simulink model "gm_soc_dvbs2_fpga"  (R2025b)
settings: Solver=VariableStepAuto  StartTime=0.0  StopTime=10.0  RelTol=1e-3
InitFcn:
  | soc_dvbs2_init;
undefined symbols (not defined in the file or in its folder): Add, coefficientsLog, coefficientsSqrt1, coefficientsSqrt2, dataBits, Deinterleaver, designMultirateFIR, noisePow, Shift, Short, soc_dvbs2_designFIRFilter, soc_dvbs2_txPacketBits, syncWord, txDataOut, txFiltCoeff, XData
libraries: simulink x304, hdlsllib x265, dspsigops x15, dsphdlfiltering2 x8, hdlmdlgenlib x6, dsphdlsigops2 x5, commseqgen3 x5, dsphdlmathfun2 x3, hwlogicconnlib x2, whdledac x2, commhdlcrc x2, whdlutilities x1
(part 8 of 36)

== system gm_soc_dvbs2_fpga/DVBS2/DVBS2 TxRx/Channel/AWGN Generator/Unit Variance Gaussian Noise/SinCos ==
  u1 : Inport  OutDataTypeStr=fixdt(0, 16, 16)  PortDimensions=1  SampleTime=6.25e-08
  Delay : Delay  DelayLength=double(1)  InitialCondition=0  SampleTime=6.25e-08
  Delay1 : Delay  DelayLength=double(1)  InitialCondition=0  SampleTime=6.25e-08
  Delay3 : Delay  DelayLength=double(1)  InitialCondition=0  SampleTime=6.25e-08
  Sine HDL Optimized1 : Subsystem  mask(Sine and Cosine HDL optimized block){OutputFormula=cos(2*pi*u), NumDataPoints=double(1024), TableDataTypeStr=fixdt(0,15,15), SimulateLUTROMDelay=off}
      mask prompts: OutputFormula "Simulink:masks:OutputFormula_MP"; NumDataPoints "HDLShared:hdlshared:CosineHDL_Npts"; TableDataTypeStr "Simulink:blkprm_prompts:TABLE_UNIFIEDDATATYPE"; SimulateLUTROMDelay "HDLShared:hdlshared:CosineHDL_SimulateLUTDelay"
      mask help: Sine and Cosine HDL optimized block using quarter wave symmetry, and HDL friendly settings.
      mask init:
      | NumDataPoints = double(1024);
      | OutputFormula = double(2);
      | SampleTime = double(-1);
      | SimulateLUTROMDelay = double(0);
      | TableDataTypeStr = fixdt(0,15,15);
      | curr_blk_name = 'soc_dvbs2_fpga/DVBS2/DVBS2 TxRx/Channel/AWGN Generator/Unit Variance Gaussian Noise/SinCos/Sine\nHDL Optimized1';
      | sys_name = 'soc_dvbs2_fpga/DVBS2/DVBS2 TxRx/Channel/AWGN Generator/Unit Variance Gaussian Noise/SinCos';
      mask Help: helpview([docroot '/hdlcoder/helptargets.map'],'SineAndCosineHDL_Optimized');
      mask TypeOptions OutputFormula: sin(2*pi*u) | cos(2*pi*u) | exp(j*2*pi*u) | sin(2*pi*u) and cos(2*pi*u)
      mask Display:
      | port_label('input',1,'u')
      | port_label('output',1,'cos(2*pi*u)')
      | xpos = 0.35;
      | yoffset = 0.5;
      | if ( SimulateLUTROMDelay )
      |   text(xpos,yoffset,'HDL (Z^{-1})','texmode','on')
      | else
      |    text(xpos,yoffset,'HDL')
      | end
  Sine HDL Optimized2 : Subsystem  mask(Sine and Cosine HDL optimized block){OutputFormula=sin(2*pi*u), NumDataPoints=double(1024), TableDataTypeStr=fixdt(0,15,15), SimulateLUTROMDelay=off}
      mask prompts: OutputFormula "Simulink:masks:OutputFormula_MP"; NumDataPoints "HDLShared:hdlshared:CosineHDL_Npts"; TableDataTypeStr "Simulink:blkprm_prompts:TABLE_UNIFIEDDATATYPE"; SimulateLUTROMDelay "HDLShared:hdlshared:CosineHDL_SimulateLUTDelay"
      mask help: Sine and Cosine HDL optimized block using quarter wave symmetry, and HDL friendly settings.
      mask init:
      | NumDataPoints = double(1024);
      | OutputFormula = double(1);
      | SampleTime = double(-1);
      | SimulateLUTROMDelay = double(0);
      | TableDataTypeStr = fixdt(0,15,15);
      | curr_blk_name = 'soc_dvbs2_fpga/DVBS2/DVBS2 TxRx/Channel/AWGN Generator/Unit Variance Gaussian Noise/SinCos/Sine\nHDL Optimized2';
      | sys_name = 'soc_dvbs2_fpga/DVBS2/DVBS2 TxRx/Channel/AWGN Generator/Unit Variance Gaussian Noise/SinCos';
      mask Help: helpview([docroot '/hdlcoder/helptargets.map'],'SineAndCosineHDL_Optimized');
      mask TypeOptions OutputFormula: sin(2*pi*u) | cos(2*pi*u) | exp(j*2*pi*u) | sin(2*pi*u) and cos(2*pi*u)
      mask Display:
      | port_label('input',1,'u')
      | port_label('output',1,'sin(2*pi*u)')
      | xpos = 0.35;
      | yoffset = 0.5;
      | if ( SimulateLUTROMDelay )
      |   text(xpos,yoffset,'HDL (Z^{-1})','texmode','on')
      | else
      |    text(xpos,yoffset,'HDL')
      | end
  g0 : Outport  SampleTime=6.25e-08
  g1(16,15) : Outport  Port=2  SampleTime=6.25e-08
  wires:
  Sine HDL Optimized1/1(x) -> Delay1/1
  u1/1 -> Delay3/1
  Delay3/1 -> Sine HDL Optimized2/1(u), Sine HDL Optimized1/1(u)
  Sine HDL Optimized2/1(x) -> Delay/1
  Delay1/1 -> g1(16,15)/1
  Delay/1 -> g0/1

== system gm_soc_dvbs2_fpga/DVBS2/DVBS2 TxRx/Channel/AWGN Generator/Unit Variance Gaussian Noise/SqrtImplementation ==
  u : Inport  OutDataTypeStr=fixdt(0, 31, 24)  PortDimensions=1  SampleTime=6.25e-08
  Constant : Constant  Value=0  OutDataTypeStr=fixdt(0,17,13)  SampleTime=-1
  Delay : Delay  DelayLength=19
  Delay1 : Delay  DelayLength=19
  SqrtEval : Subsystem
  Switch : Switch  Criteria=u2 ~= 0  OutDataTypeStr=fixdt(0, 17, 13)  SaturateOnIntegerOverflow=off  InputSameDT=off
  f : Outport  SampleTime=6.25e-08  VectorParamsAs1DForOutWhenUnconnected=off
  wires:
  u/1 -> Delay/1, SqrtEval/1(u)
  Switch/1 -> f/1
  Delay/1 -> Switch/2
  Constant/1 -> Delay1/1
  Delay1/1 -> Switch/3
  SqrtEval/1(f) -> Switch/1

== system gm_soc_dvbs2_fpga/DVBS2/DVBS2 TxRx/Channel/AWGN Generator/Unit Variance Gaussian Noise/TausUniformRandGen ==
  ConcatandExtract : Subsystem
  TausURNG1 : Subsystem
  TausURNG2 : Subsystem
  u0(16,16) : Outport  SampleTime=6.25e-08
  u1(16,16) : Outport  Port=2  SampleTime=6.25e-08
  wires:
  TausURNG1/1(a) -> ConcatandExtract/1(a)
  TausURNG2/1(b) -> ConcatandExtract/2(b)
  ConcatandExtract/2(u1(16,16)) -> u1(16,16)/1
  ConcatandExtract/1(u0(48,48)) -> u0(16,16)/1

== system gm_soc_dvbs2_fpga/DVBS2/DVBS2 TxRx/Channel/AWGN Generator/Unit Variance Gaussian Noise/logImplementation ==
  u0(48,48) : Inport  OutDataTypeStr=fixdt(0, 48, 48)  PortDimensions=1  SampleTime=6.25e-08
  Constant : Constant  Value=0  OutDataTypeStr=fixdt(0,16,9)  SampleTime=-1
  Delay : Delay  DelayLength=24
  Switch : Switch  Criteria=u2 ~= 0  OutDataTypeStr=fixdt(0, 31, 24)  SaturateOnIntegerOverflow=off  InputSameDT=off
  log : Subsystem
  e : Outport  SampleTime=6.25e-08
  wires:
  u0(48,48)/1 -> Delay/1, log/1(u0(48,48))
  log/1(e) -> Switch/1
  Switch/1 -> e/1
  Constant/1 -> Switch/3
  Delay/1 -> Switch/2

== system gm_soc_dvbs2_fpga/DVBS2/DVBS2 TxRx/DVB-S2 HDL Receiver/Demod Deinterleave and FECDecode/DVBS2 HDL Deinterleaver/Discard Out of  Frame samples ==
  dataIn : Inport  OutDataTypeStr=fixdt(1, 8, 4)  PortDimensions=1  SampleTime=7.8125e-09
  valid : Inport  Port=2  OutDataTypeStr=boolean  PortDimensions=1  SampleTime=7.8125e-09
  reset : Inport  Port=3  OutDataTypeStr=boolean  PortDimensions=1  SampleTime=7.8125e-09
  fec : Inport  Port=4  OutDataTypeStr=boolean  PortDimensions=1  SampleTime=7.8125e-09
  Discard Out of  Frame samples : MATLAB Function  TreatAsAtomicUnit=on
  dataOut : Outport  SampleTime=7.8125e-09
  validOut : Outport  Port=2  SampleTime=7.8125e-09
  wires:
  reset/1 -> Discard Out of  Frame samples/3(reset)
  dataIn/1 -> Discard Out of  Frame samples/1(dataIn)
  valid/1 -> Discard Out of  Frame samples/2(valid)
  fec/1 -> Discard Out of  Frame samples/4(fec)
  Discard Out of  Frame samples/2(validOut) -> validOut/1
  Discard Out of  Frame samples/1(dataOut) -> dataOut/1

== system gm_soc_dvbs2_fpga/DVBS2/DVBS2 TxRx/DVB-S2 HDL Receiver/Demod Deinterleave and FECDecode/DVBS2 HDL Deinterleaver/RAM ==
  wr_din : Inport  OutDataTypeStr=fixdt(1, 8, 4)  PortDimensions=1  SampleTime=7.8125e-09
  wr_addr : Inport  Port=2  OutDataTypeStr=fixdt(0, 17, 0)  PortDimensions=1  SampleTime=7.8125e-09
  wr_en : Inport  Port=3  OutDataTypeStr=boolean  PortDimensions=1  SampleTime=7.8125e-09
  rd_addr : Inport  Port=4  OutDataTypeStr=fixdt(0, 18, 0)  PortDimensions=1  SampleTime=7.8125e-09
  rd_valid : Inport  Port=5  OutDataTypeStr=boolean  PortDimensions=1  SampleTime=7.8125e-09
  rd_end : Inport  Port=6  OutDataTypeStr=boolean  PortDimensions=1  SampleTime=7.8125e-09
  rd_start : Inport  Port=7  OutDataTypeStr=boolean  PortDimensions=1  SampleTime=7.8125e-09
  Delay : Delay  DelayLength=1
  Delay1 : Delay  DelayLength=1
  Delay{3..13} (11 alike) : Delay
  Delay2 : Delay  DelayLength=1
  Single RAM Using Two RAMs : Subsystem
  Wrap Address : Subsystem
  rd_dout : Outport  SampleTime=7.8125e-09
  rd_startOut : Outport  Port=2  SampleTime=7.8125e-09
  rd_endOut : Outport  Port=3  SampleTime=7.8125e-09
  rd_validOut : Outport  Port=4  SampleTime=7.8125e-09
  wires:
  rd_end/1 -> Delay5/1
  rd_start/1 -> Delay4/1
  rd_addr/1 -> Wrap Address/1(u)
  rd_valid/1 -> Delay3/1
  Delay3/1 -> Delay/1
  wr_en/1 -> Delay7/1
  wr_addr/1 -> Delay6/1
  wr_din/1 -> Delay12/1
  Wrap Address/1(y) -> Delay8/1
  Delay4/1 -> Delay1/1
  Delay5/1 -> Delay2/1
  Delay/1 -> Delay10/1
  Delay11/1 -> rd_startOut/1
  Delay7/1 -> Single RAM Using Two RAMs/3(wr_en)
  Delay12/1 -> Single RAM Using Two RAMs/1(wr_din)
  Delay6/1 -> Single RAM Using Two RAMs/2(wr_addr)
  Delay8/1 -> Single RAM Using Two RAMs/4(rd_addr)
  Delay1/1 -> Delay11/1
  Delay2/1 -> Delay13/1
  Delay10/1 -> rd_validOut/1
  Single RAM Using Two RAMs/1(rd_dout) -> Delay9/1
  Delay13/1 -> rd_endOut/1
  Delay9/1 -> rd_dout/1

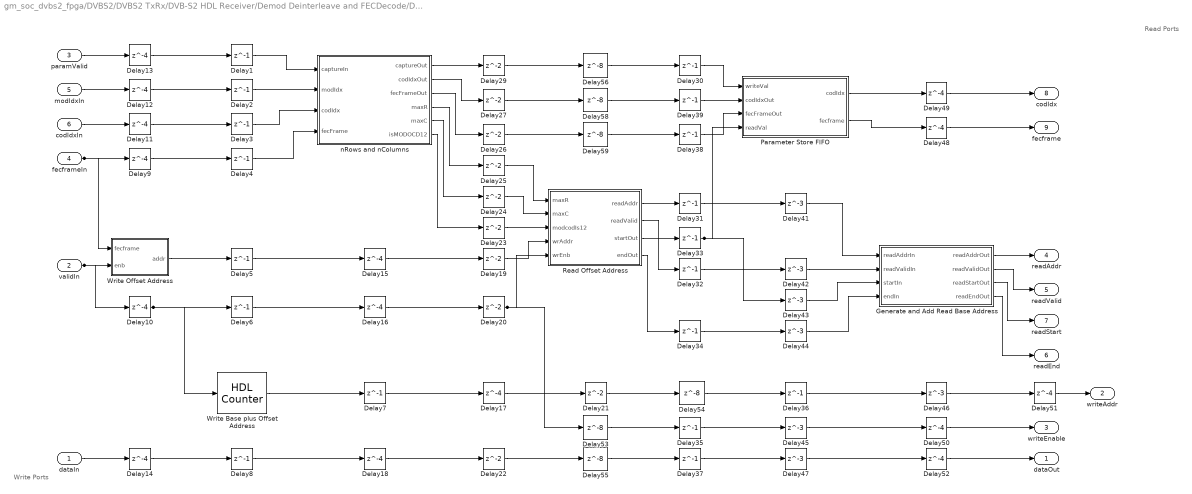
== system gm_soc_dvbs2_fpga/DVBS2/DVBS2 TxRx/DVB-S2 HDL Receiver/Demod Deinterleave and FECDecode/DVBS2 HDL Deinterleaver/RAM Address Generator ==
  note: Read Ports
  note: Write Ports
  dataIn : Inport  OutDataTypeStr=fixdt(1, 8, 4)  PortDimensions=1  SampleTime=7.8125e-09
  validIn : Inport  Port=2  OutDataTypeStr=boolean  PortDimensions=1  SampleTime=7.8125e-09
  paramValid : Inport  Port=3  OutDataTypeStr=boolean  PortDimensions=1  SampleTime=7.8125e-09
  fecframeIn : Inport  Port=4  OutDataTypeStr=boolean  PortDimensions=1  SampleTime=7.8125e-09
  modIdxIn : Inport  Port=5  OutDataTypeStr=fixdt(0, 2, 0)  PortDimensions=1  SampleTime=7.8125e-09
  codIdxIn : Inport  Port=6  OutDataTypeStr=fixdt(0, 4, 0)  PortDimensions=1  SampleTime=7.8125e-09
  Delay{1..8,30..39} (18 alike) : Delay  DelayLength=1
  Delay{9..18,48..52} (15 alike) : Delay  DelayLength=4
  Delay{19..27,29} (10 alike) : Delay
  Delay{41..47} (7 alike) : Delay  DelayLength=3
  Delay{53..56,58..59} (6 alike) : Delay  DelayLength=8
  Generate and Add Read Base Address : Subsystem
  Parameter Store FIFO : Subsystem
  Read Offset Address : Subsystem
  Write Base plus Offset Address : hdlsllib/Sources/HDL Counter  CountType=Count limited  CountInit=0  CountStep=1  CountMax=ConfigRx.RAMCapacity - 1  CountFromType=Initial value  CountFrom=0  CountResetPort=off  CountLoadPort=off  CountEnbPort=on  CountDirPort=off  CountHitOutputPort=off  CountDataType=Unsigned  CountWordLen=nextpow2(ConfigRx.RAMCapacity - 1)  CountFracLen=0  CountSampTime=1
  Write Offset Address : Subsystem
  nRows and nColumns : Subsystem
  dataOut : Outport  SampleTime=7.8125e-09
  writeAddr : Outport  Port=2  SampleTime=7.8125e-09
  writeEnable : Outport  Port=3  SampleTime=7.8125e-09
  readAddr : Outport  Port=4  SampleTime=7.8125e-09
  readValid : Outport  Port=5  SampleTime=7.8125e-09
  readEnd : Outport  Port=6  SampleTime=7.8125e-09
  readStart : Outport  Port=7  SampleTime=7.8125e-09
  codIdx : Outport  Port=8  SampleTime=7.8125e-09
  fecframe : Outport  Port=9  SampleTime=7.8125e-09
  wires:
  dataIn/1 -> Delay14/1
  Delay26/1 -> Delay59/1
  nRows and nColumns/2(codIdxOut) -> Delay27/1
  Delay33/1 -> Parameter Store FIFO/4(readVal), Delay43/1
  Delay25/1 -> Read Offset Address/1(maxR)
  nRows and nColumns/3(fecFrameOut) -> Delay26/1
  validIn/1 -> Delay10/1, Write Offset Address/2(enb)
  Delay31/1 -> Delay41/1
  nRows and nColumns/1(captureOut) -> Delay29/1
  fecframeIn/1 -> Delay9/1, Write Offset Address/1(fecframe)
  Delay3/1 -> nRows and nColumns/3(codIdx)
  codIdxIn/1 -> Delay11/1
  modIdxIn/1 -> Delay12/1
  Delay30/1 -> Parameter Store FIFO/1(writeVal)
  Delay32/1 -> Delay42/1
  Delay24/1 -> Read Offset Address/2(maxC)
  paramValid/1 -> Delay13/1
  Delay12/1 -> Delay2/1
  Write Base plus Offset Address/1 -> Delay7/1
  Delay13/1 -> Delay1/1
  Delay11/1 -> Delay3/1
  Delay9/1 -> Delay4/1
  Delay55/1 -> Delay37/1
  Write Offset Address/1(addr) -> Delay5/1
  Delay10/1 -> Write Base plus Offset Address/1, Delay6/1
  Delay14/1 -> Delay8/1
  Delay1/1 -> nRows and nColumns/1(captureIn)
  Delay19/1 -> Read Offset Address/4(wrAddr)
  Delay2/1 -> nRows and nColumns/2(modIdx)
  Delay4/1 -> nRows and nColumns/4(fecFrame)
  Delay5/1 -> Delay15/1
  Delay6/1 -> Delay16/1
  Delay8/1 -> Delay18/1
  Delay29/1 -> Delay56/1
  nRows and nColumns/4(maxR) -> Delay25/1
  Delay27/1 -> Delay58/1
  nRows and nColumns/5(maxC) -> Delay24/1
  nRows and nColumns/6(isMODOCD12) -> Delay23/1
  Delay23/1 -> Read Offset Address/3(modcodIs12)
  Delay15/1 -> Delay19/1
  Delay16/1 -> Delay20/1
  Delay7/1 -> Delay17/1
  Delay22/1 -> Delay55/1
  Delay18/1 -> Delay22/1
  Delay20/1 -> Delay53/1, Read Offset Address/5(wrEnb)
  Delay17/1 -> Delay21/1
  Delay21/1 -> Delay54/1
  Delay56/1 -> Delay30/1
  Delay58/1 -> Delay39/1
  Delay59/1 -> Delay38/1
  Read Offset Address/1(readAddr) -> Delay31/1
  Read Offset Address/2(readValid) -> Delay32/1
  Read Offset Address/3(startOut) -> Delay33/1
  Read Offset Address/4(endOut) -> Delay34/1
  Delay53/1 -> Delay35/1
  Delay39/1 -> Parameter Store FIFO/2(codIdxOut)
  Delay38/1 -> Parameter Store FIFO/3(fecFrameOut)
  Delay34/1 -> Delay44/1
  Delay54/1 -> Delay36/1
  Delay35/1 -> Delay45/1
  Delay37/1 -> Delay47/1
  Parameter Store FIFO/1(codIdx) -> Delay49/1
  Parameter Store FIFO/2(fecframe) -> Delay48/1
  Delay41/1 -> Generate and Add Read Base Address/1(readAddrIn)
  Delay42/1 -> Generate and Add Read Base Address/2(readValidIn)
  Delay43/1 -> Generate and Add Read Base Address/3(startIn)
  Delay44/1 -> Generate and Add Read Base Address/4(endIn)
  Delay36/1 -> Delay46/1
  Delay45/1 -> Delay50/1
  Delay47/1 -> Delay52/1
  Delay49/1 -> codIdx/1
  Delay48/1 -> fecframe/1
  Generate and Add Read Base Address/1(readAddrOut) -> readAddr/1
  Generate and Add Read Base Address/2(readValidOut) -> readValid/1
  Generate and Add Read Base Address/3(readStartOut) -> readStart/1
  Generate and Add Read Base Address/4(readEndOut) -> readEnd/1
  Delay46/1 -> Delay51/1
  Delay50/1 -> writeEnable/1
  Delay52/1 -> dataOut/1
  Delay51/1 -> writeAddr/1

== system gm_soc_dvbs2_fpga/DVBS2/DVBS2 TxRx/DVB-S2 HDL Receiver/Demod Deinterleave and FECDecode/Discard Unsupported Frames/convertMODCOD ==
  modcod : Inport  OutDataTypeStr=fixdt(0, 5, 0)  PortDimensions=1  SampleTime=7.8125e-09
  convertMODCOD : MATLAB Function  TreatAsAtomicUnit=on
  modIdx : Outport  SampleTime=7.8125e-09
  codIdx : Outport  Port=2  SampleTime=7.8125e-09
  wires:
  modcod/1 -> convertMODCOD/1(modcod)
  convertMODCOD/2(codIdx) -> codIdx/1
  convertMODCOD/1(modIdx) -> modIdx/1

== system gm_soc_dvbs2_fpga/DVBS2/DVBS2 TxRx/DVB-S2 HDL Receiver/Stream Recovery/BB Decoder/Extract BBHeader ==
  bitsIn : Inport  OutDataTypeStr=boolean  PortDimensions=1  SampleTime=7.8125e-09
  reset : Inport  Port=2  OutDataTypeStr=boolean  PortDimensions=1  SampleTime=7.8125e-09
  validIn : Inport  Port=3  OutDataTypeStr=boolean  PortDimensions=1  SampleTime=7.8125e-09
  Bit Index : hdlsllib/Sources/HDL Counter  CountType=Count limited  CountInit=0  CountStep=1  CountMax=80 - 8 - 1  CountFromType=Initial value  CountFrom=0  CountResetPort=on  CountLoadPort=off  CountEnbPort=on  CountDirPort=off  CountHitOutputPort=off  CountDataType=Unsigned  CountWordLen=nextpow2(80 - 8 - 1)  CountFracLen=0  CountSampTime=1
  Extract DFL : Subsystem
  Extract MATYPE1 : Subsystem
  Extract MATYPE2 : Subsystem
  Extract SYNC : Subsystem
  Extract SYNCD : Subsystem
  Extract UPL : Subsystem
  Saturate UPL value : Subsystem
  TSorGS : Outport  SampleTime=7.8125e-09
  SISorMIS : Outport  Port=2  SampleTime=7.8125e-09
  CCMorACM : Outport  Port=3  SampleTime=7.8125e-09
  ISSYI : Outport  Port=4  SampleTime=7.8125e-09
  NPD : Outport  Port=5  SampleTime=7.8125e-09
  RO : Outport  Port=6  SampleTime=7.8125e-09
  MIS_ISI : Outport  Port=7  SampleTime=7.8125e-09
  UPL : Outport  Port=8  SampleTime=7.8125e-09
  DFL : Outport  Port=9  SampleTime=7.8125e-09
  SYNC : Outport  Port=10  SampleTime=7.8125e-09
  SYNCD : Outport  Port=11  SampleTime=7.8125e-09
  wires:
  reset/1 -> Bit Index/1
  Extract MATYPE1/3(CCMorACM) -> CCMorACM/1
  Extract MATYPE1/1(TSorGS) -> TSorGS/1
  validIn/1 -> Extract MATYPE1/3(validIn), Extract MATYPE2/3(validIn), Extract DFL/3(validIn), Extract SYNC/3(validIn), Extract SYNCD/3(validIn), Bit Index/2, Extract UPL/3(validIn)
  Extract MATYPE2/1(MIS_ISI) -> MIS_ISI/1
  Extract MATYPE1/2(SISorMIS) -> SISorMIS/1
  Extract MATYPE1/4(ISSYI) -> ISSYI/1
  Bit Index/1 -> Extract MATYPE1/2(idx), Extract MATYPE2/2(idx), Extract UPL/2(idx), Extract DFL/2(idx), Extract SYNC/2(idx), Extract SYNCD/2(idx)
  bitsIn/1 -> Extract UPL/1(bitsIn), Extract SYNC/1(bitsIn), Extract SYNCD/1(bitsIn), Extract MATYPE1/1(bitsIn), Extract DFL/1(bitsIn), Extract MATYPE2/1(bitsIn)
  Extract MATYPE1/5(NPD) -> NPD/1
  Extract MATYPE1/6(RO) -> RO/1
  Extract SYNC/1(SYNC) -> SYNC/1
  Extract DFL/1(DFL) -> Saturate UPL value/2(DFL), DFL/1
  Extract UPL/1(UPL) -> Saturate UPL value/1(UPL)
  Extract SYNCD/1(DFL) -> SYNCD/1
  Saturate UPL value/1(saturatedUPL) -> UPL/1

== system gm_soc_dvbs2_fpga/DVBS2/DVBS2 TxRx/DVB-S2 HDL Receiver/Stream Recovery/BB Decoder/Extract Data Field ==
  dataIn : Inport  OutDataTypeStr=boolean  PortDimensions=1  SampleTime=7.8125e-09
  startIn : Inport  Port=2  OutDataTypeStr=boolean  PortDimensions=1  SampleTime=7.8125e-09
  validIn : Inport  Port=3  OutDataTypeStr=boolean  PortDimensions=1  SampleTime=7.8125e-09
  DFL : Inport  Port=4  OutDataTypeStr=uint16  PortDimensions=1  SampleTime=7.8125e-09
  Delay{2,19..21} (4 alike) : Delay  DelayLength=1
  Indicate SYNCD bit : Subsystem
  Sample Discard Control : Subsystem
  dataOut : Outport  SampleTime=7.8125e-09
  startOut : Outport  Port=2  SampleTime=7.8125e-09
  endOut : Outport  Port=3  SampleTime=7.8125e-09
  validOut : Outport  Port=4  SampleTime=7.8125e-09
  wires:
  Delay20/1 -> Sample Discard Control/2(startIn)
  startIn/1 -> Delay20/1, Indicate SYNCD bit/1(rst)
  DFL/1 -> Delay2/1
  Delay21/1 -> Indicate SYNCD bit/3(validIn), Sample Discard Control/4(validIn)
  dataIn/1 -> Delay19/1
  validIn/1 -> Delay21/1
  Sample Discard Control/4(validOut) -> validOut/1
  Delay2/1 -> Indicate SYNCD bit/2(Distance)
  Delay19/1 -> Sample Discard Control/1(dataIn)
  Indicate SYNCD bit/1(trigger) -> Sample Discard Control/3(endIn)
  Sample Discard Control/1(dataOut) -> dataOut/1
  Sample Discard Control/2(startOut) -> startOut/1
  Sample Discard Control/3(endOut) -> endOut/1

== system gm_soc_dvbs2_fpga/DVBS2/DVBS2 TxRx/DVB-S2 HDL Receiver/Stream Recovery/BB Decoder/Extract Stream ==
  bitsIn : Inport  OutDataTypeStr=boolean  PortDimensions=1  SampleTime=7.8125e-09
  startIn : Inport  Port=2  OutDataTypeStr=boolean  PortDimensions=1  SampleTime=7.8125e-09
  endIn : Inport  Port=3  OutDataTypeStr=boolean  PortDimensions=1  SampleTime=7.8125e-09
  validIn : Inport  Port=4  OutDataTypeStr=boolean  PortDimensions=1  SampleTime=7.8125e-09
  UPL : Inport  Port=5  OutDataTypeStr=uint16  PortDimensions=1  SampleTime=7.8125e-09
  SYNC : Inport  Port=6  OutDataTypeStr=uint8  PortDimensions=1  SampleTime=7.8125e-09
  SYNCD : Inport  Port=7  OutDataTypeStr=uint16  PortDimensions=1  SampleTime=7.8125e-09
  Constant1 : Constant  Value=0  OutDataTypeStr=boolean  SampleTime=-1
  Delay{,1..4,11} (6 alike) : Delay  DelayLength=3
  Delay10 : Delay  DelayLength=26-8
  Delay{5..9,12} (6 alike) : Delay  DelayLength=26
  Delay{13..17} (5 alike) : Delay
  "Extract User Packet " : Subsystem
  Insert SYNC : Subsystem
  Switch{,1..3,5} (5 alike) : Switch  Criteria=u2 ~= 0  OutDataTypeStr=boolean  SaturateOnIntegerOverflow=off  InputSameDT=off
  User Packet CRC Check : commhdlcrc/General CRC Syndrome Detector HDL Optimized  Polynomial=[1 1 1 0 1 0 1 0 1]  InitialState=0  DirectMethod=off  ReflectInput=off  ReflectCRCChecksum=off  FinalXORValue=0  SimulateUsing=Code generation
  User Packet CRC Check_term4 : Terminator
  bitsOut : Outport  SampleTime=7.8125e-09
  startOut : Outport  Port=2  SampleTime=7.8125e-09
  endOut : Outport  Port=3  SampleTime=7.8125e-09
  validOut : Outport  Port=4  SampleTime=7.8125e-09
  invalidPkt : Outport  Port=5  SampleTime=7.8125e-09
  wires:
  User Packet CRC Check/2 -> Insert SYNC/3(startIn)
  Delay6/1 -> Delay14/1
  validIn/1 -> Delay3/1, "Extract User Packet "/5(validIn)
  Delay8/1 -> Delay16/1
  startIn/1 -> Delay1/1, "Extract User Packet "/3(startIn)
  Delay16/1 -> Switch3/3
  SYNCD/1 -> "Extract User Packet "/1(SYNCD)
  Delay13/1 -> Switch/3
  UPL/1 -> Delay4/1, "Extract User Packet "/6(UPL)
  Delay9/1 -> Delay17/1
  SYNC/1 -> Delay11/1
  Delay15/1 -> Switch2/3
  endIn/1 -> Delay2/1, "Extract User Packet "/4(endIn)
  Delay17/1 -> Switch5/2, Switch2/2, Switch1/2, Switch3/2, Switch/2
  User Packet CRC Check/3 -> Insert SYNC/4(endIn)
  bitsIn/1 -> Delay/1, "Extract User Packet "/2(bitsIn)
  Delay1/1 -> Delay6/1
  "Extract User Packet "/1(dataOut) -> User Packet CRC Check/1
  "Extract User Packet "/2(startOut) -> User Packet CRC Check/2
  "Extract User Packet "/3(endOut) -> User Packet CRC Check/3
  Switch1/1 -> startOut/1
  "Extract User Packet "/4(validOut) -> User Packet CRC Check/4
  "Extract User Packet "/5(invalidPkt) -> Delay10/1
  Delay11/1 -> Delay12/1
  Delay12/1 -> Insert SYNC/6(SYNC)
  User Packet CRC Check/4 -> Insert SYNC/5(validIn)
  Delay4/1 -> Delay9/1
  Delay2/1 -> Delay7/1
  Delay/1 -> Delay5/1
  Delay3/1 -> Delay8/1
  Delay10/1 -> Insert SYNC/1(invalidIn)
  User Packet CRC Check/1 -> Insert SYNC/2(dataIn)
  Delay7/1 -> Delay15/1
  User Packet CRC Check/5 -> User Packet CRC Check_term4/1
  Delay5/1 -> Delay13/1
  Delay14/1 -> Switch1/3
  Constant1/1 -> Switch5/3
  Insert SYNC/1(invalidOut) -> Switch5/1
  Insert SYNC/2(dataOut) -> Switch/1
  Insert SYNC/3(startOut) -> Switch1/1
  Insert SYNC/4(endOut) -> Switch2/1
  Insert SYNC/5(validOut) -> Switch3/1
  Switch5/1 -> invalidPkt/1
  Switch2/1 -> endOut/1
  Switch/1 -> bitsOut/1
  Switch3/1 -> validOut/1

== system gm_soc_dvbs2_fpga/DVBS2/DVBS2 TxRx/DVB-S2 HDL Receiver/Stream Recovery/BB Descrambler/Subsystem ==
  In1 : Inport  OutDataTypeStr=boolean  PortDimensions=1  SampleTime=7.8125e-09
  Enable : EnablePort  OutDataTypeStr=boolean
  PN Sequence Generator : commseqgen3/PN Sequence Generator  poly='z^15 + z + 1'  ini_sta=[1 0 0 1 0 1 0 1 0 0 0 0 0 0 0]  outBitMaskSource=Dialog parameter  shift=15  outVarSiz=off  maxOutSizeMode=Dialog parameter  maxOutSize=[10 1]  Ts=-1  sampPerFrame=1  reset=on  bitPackedOutputs=off  outDataType=Smallest unsigned integer  numPackedBits=8  bitPackDataSigned=off  bitPackedOutDType=double
  Out1 : Outport  SampleTime=7.8125e-09  InitialOutput=0
  wires:
  PN Sequence Generator/1 -> Out1/1
  In1/1 -> PN Sequence Generator/1

== system gm_soc_dvbs2_fpga/DVBS2/DVBS2 TxRx/DVB-S2 HDL Receiver/Stream Recovery/BB Header CRC Check/Discard CRC failed Frame ==
  startIn : Inport  OutDataTypeStr=boolean  PortDimensions=1  SampleTime=7.8125e-09
  validIn : Inport  Port=2  OutDataTypeStr=boolean  PortDimensions=1  SampleTime=7.8125e-09
  bitsIn : Inport  Port=3  OutDataTypeStr=boolean  PortDimensions=1  SampleTime=7.8125e-09
  err : Inport  Port=4  OutDataTypeStr=boolean  PortDimensions=1  SampleTime=7.8125e-09
  errorValid : Inport  Port=5  OutDataTypeStr=boolean  PortDimensions=1  SampleTime=7.8125e-09
  Delay10 : Delay  DelayLength=1
  Delay12 : Delay  DelayLength=1
  Delay9 : Delay  DelayLength=1
  Logical Operator : Logic  Operator=NOT  AllPortsSameDT=off  OutDataTypeStr=boolean
  Logical Operator1 : Logic  AllPortsSameDT=off  OutDataTypeStr=boolean
  Logical Operator2 : Logic  AllPortsSameDT=off  OutDataTypeStr=boolean
  Logical Operator4 : Logic  AllPortsSameDT=off  OutDataTypeStr=boolean
  Unit Delay Enabled Resettable Synchronous : hdlsllib/Discrete/Unit Delay Enabled Resettable Synchronous  InitialCondition=0.0  SampleTime=-1
  startOut : Outport  SampleTime=7.8125e-09
  validOut : Outport  Port=2  SampleTime=7.8125e-09
  bitsOut : Outport  Port=3  SampleTime=7.8125e-09
  wires:
  validIn/1 -> Delay10/1
  err/1 -> Unit Delay Enabled Resettable Synchronous/3, Logical Operator/1
  errorValid/1 -> Unit Delay Enabled Resettable Synchronous/2
  bitsIn/1 -> Delay9/1
  startIn/1 -> Delay12/1
  Delay12/1 -> Logical Operator4/1
  Logical Operator/1 -> Unit Delay Enabled Resettable Synchronous/1
  Delay9/1 -> Logical Operator1/1
  Unit Delay Enabled Resettable Synchronous/1 -> Logical Operator4/2, Logical Operator2/2, Logical Operator1/2
  Delay10/1 -> Logical Operator2/1
  Logical Operator4/1 -> startOut/1
  Logical Operator1/1 -> bitsOut/1
  Logical Operator2/1 -> validOut/1

== system gm_soc_dvbs2_fpga/DVBS2/DVBS2 TxRx/DVB-S2 HDL Receiver/Synchronizer and PL Header Decoder/Fine Phase Synchronizer/Direct Digital Synthesis ==
  v : Inport  OutDataTypeStr=fixdt(1, 21, 21)  PortDimensions=1  SampleTime=2.5e-07
  rst : Inport  Port=2  OutDataTypeStr=boolean  PortDimensions=1  SampleTime=2.5e-07
  Constant : Constant  Value=true  OutDataTypeStr=boolean  SampleTime=-1
  Constant1 : Constant  Value=FPCV  OutDataTypeStr=boolean  SampleTime=-1
  Constant2 : Constant  Value=complex(1)  OutDataTypeStr=fixdt(1, 16, 14)  SampleTime=-1
  Data Type Conversion : DataTypeConversion  OutDataTypeStr=fixdt(1,21,21)  SaturateOnIntegerOverflow=off  RndMeth=Floor
  Data Type Conversion1 : DataTypeConversion  OutDataTypeStr=fixdt(1,21,0)  ConvertRealWorld=Stored Integer (SI)  SaturateOnIntegerOverflow=off  RndMeth=Floor
  Delay1 : Delay  DelayLength=1
  Delay12 : Delay  DelayLength=1
  Multiport Switch : MultiPortSwitch  DataPortOrder=Zero-based contiguous  Inputs=2  zeroidx=on  OutDataTypeStr=fixdt(1, 16, 14)  SaturateOnIntegerOverflow=off  InputSameDT=off
  NCO HDL Optimized : dsphdlsigops2/NCO  PhaseIncrementSource=Property  PhaseIncrement=0  PhaseOffsetSource=Input port  PhaseOffset=0  DitherSource=None  NumDitherBits=4  SamplesPerFrame=1  LUTCompress=off  ResetAction=on  Waveform=Complex exponential  PhasePort=off  SimulateUsing=Code generation  AccumulatorWL=21  PhaseQuantization=on  NumQuantizerAccumulatorBits=14  OutputDataType=Binary point scaling  OutputWL=16  OutputFL=14
  NCO HDL Optimized_term1 : Terminator
  xph : Outport  SampleTime=2.5e-07
  wires:
  v/1 -> Delay12/1
  Constant2/1 -> Multiport Switch/2
  Delay12/1 -> Data Type Conversion/1
  Constant1/1 -> Multiport Switch/1
  rst/1 -> NCO HDL Optimized/2
  Data Type Conversion/1 -> Data Type Conversion1/1
  Data Type Conversion1/1 -> NCO HDL Optimized/1
  Constant/1 -> NCO HDL Optimized/3
  NCO HDL Optimized/1 -> Multiport Switch/3
  NCO HDL Optimized/2 -> NCO HDL Optimized_term1/1
  Multiport Switch/1 -> Delay1/1
  Delay1/1 -> xph/1

== system gm_soc_dvbs2_fpga/DVBS2/DVBS2 TxRx/DVB-S2 HDL Receiver/Synchronizer and PL Header Decoder/Fine Phase Synchronizer/Loop Filter ==
  e : Inport  OutDataTypeStr=fixdt(1, 22, 14)  PortDimensions=1  SampleTime=2.5e-07
  En : Inport  Port=2  OutDataTypeStr=boolean  PortDimensions=1  SampleTime=2.5e-07
  rst : Inport  Port=3  OutDataTypeStr=boolean  PortDimensions=1  SampleTime=2.5e-07
  Add : Sum  OutDataTypeStr=fixdt(1, 21, 21)  AccumDataTypeStr=fixdt(1, 22, 21)  SampleTime=2.5e-07
  Delay1 : Delay  DelayLength=double(2)  InitialCondition=0  SampleTime=2.5e-07
  Delay12 : Delay  DelayLength=double(2)  InitialCondition=0  SampleTime=2.5e-07
  Gain : Gain  Gain="fi(0,0,16,31,\"hex\",\"d59b\")"  ParamDataTypeStr=fixdt(0, 16, 31)  OutDataTypeStr=fixdt(1, 21, 21)  SampleTime=2.5e-07
  Unit Delay Enabled Resettable Synchronous : hdlsllib/Discrete/Unit Delay Enabled Resettable Synchronous  InitialCondition=double(0)  SampleTime=-1
  v : Outport  SampleTime=2.5e-07
  rstOut : Outport  Port=2  SampleTime=2.5e-07
  wires:
  e/1 -> Delay1/1
  Add/1 -> Unit Delay Enabled Resettable Synchronous/1
  rst/1 -> rstOut/1, Unit Delay Enabled Resettable Synchronous/3
  Gain/1 -> Delay12/1
  Delay1/1 -> Gain/1
  En/1 -> Unit Delay Enabled Resettable Synchronous/2
  Delay12/1 -> Add/1
  Unit Delay Enabled Resettable Synchronous/1 -> v/1, Add/2

== system gm_soc_dvbs2_fpga/DVBS2/DVBS2 TxRx/DVB-S2 HDL Receiver/Synchronizer and PL Header Decoder/Fine Phase Synchronizer/Phase Error Detector ==
  dataIn : Inport  OutDataTypeStr=fixdt(1, 22, 14)  PortDimensions=1  SampleTime=2.5e-07
      settings: SignalType=complex
  Compare To Constant : simulink/Logic and Bit Operations/Compare To Constant  relop=>=  const=0  OutDataTypeStr=boolean
  Compare To Constant1 : simulink/Logic and Bit Operations/Compare To Constant  relop=>=  const=0  OutDataTypeStr=boolean
  Complex to Real-Imag : ComplexToRealImag
  Complex to Real-Imag1 : ComplexToRealImag  Output=Imag
  Constant : Constant  OutDataTypeStr=fixdt(1,2,0)  SampleTime=-1
  Constant1 : Constant  Value=-1  OutDataTypeStr=fixdt(1,2,0)  SampleTime=-1
  Constant2 : Constant  OutDataTypeStr=fixdt(1,2,0)  SampleTime=-1
  Delay{1..5,12} (6 alike) : Delay  DelayLength=1
  Delay6 : Delay
  Delay7 : Delay
  Delay8 : Delay
  Product : Product  OutDataTypeStr=fixdt(1, 22, 14)
  Real-Imag to Complex : RealImagToComplex
  Switch : Switch  Criteria=u2 ~= 0  OutDataTypeStr=fixdt(1, 2, 0)  SaturateOnIntegerOverflow=off  InputSameDT=off
  Switch1 : Switch  Criteria=u2 ~= 0  OutDataTypeStr=fixdt(1, 2, 0)  SaturateOnIntegerOverflow=off  InputSameDT=off
  e : Outport  SampleTime=2.5e-07
  wires:
  Delay3/1 -> Real-Imag to Complex/1
  Constant/1 -> Switch/1
  Constant1/1 -> Switch/3, Switch1/1
  Delay12/1 -> Compare To Constant/1
  dataIn/1 -> Complex to Real-Imag/1, Delay1/1
  Delay2/1 -> Compare To Constant1/1
  Delay1/1 -> Delay5/1
  Complex to Real-Imag/1 -> Delay12/1
  Complex to Real-Imag/2 -> Delay2/1
  Delay5/1 -> Delay6/1
  Compare To Constant1/1 -> Switch1/2
  Compare To Constant/1 -> Switch/2
  Constant2/1 -> Switch1/3
  Switch/1 -> Delay3/1
  Switch1/1 -> Delay4/1
  Product/1 -> Delay8/1
  Delay4/1 -> Real-Imag to Complex/2
  Delay6/1 -> Product/1
  Real-Imag to Complex/1 -> Delay7/1
  Delay7/1 -> Product/2
  Delay8/1 -> Complex to Real-Imag1/1
  Complex to Real-Imag1/1 -> e/1

== system gm_soc_dvbs2_fpga/DVBS2/DVBS2 TxRx/DVB-S2 HDL Receiver/Synchronizer and PL Header Decoder/Fine Phase Synchronizer/Power Q and Beta Offset Rotation ==
  dataIn : Inport  OutDataTypeStr=fixdt(1, 22, 14)  PortDimensions=1  SampleTime=2.5e-07
      settings: SignalType=complex
  mod : Inport  Port=2  OutDataTypeStr=fixdt(0, 2, 0)  PortDimensions=1  SampleTime=2.5e-07
  Complex Multiplier : Subsystem
  Complex Multiplier1 : Subsystem
  Complex Multiplier2 : Subsystem
  Delay{1..3,5,7,9..12,24..27,36} (14 alike) : Delay  DelayLength=1
  Delay{4,6,8,13..20} (11 alike) : Delay  DelayLength=7
  Delay{28..35} (8 alike) : Delay
  Gain : Subsystem
  Gain1 : Subsystem
  Multiport Switch : MultiPortSwitch  DataPortOrder=Zero-based contiguous  Inputs=4  zeroidx=on  OutDataTypeStr=fixdt(1, 22, 14)  SaturateOnIntegerOverflow=off  InputSameDT=off
  dataOut : Outport  SampleTime=2.5e-07
  wires:
  Delay32/1 -> Delay19/1
  dataIn/1 -> Delay4/1, Delay6/1, Delay8/1, Complex Multiplier/1(In1), Complex Multiplier/2(In2)
  mod/1 -> Multiport Switch/1
  Delay8/1 -> Delay7/1
  Multiport Switch/1 -> Delay36/1
  Delay6/1 -> Delay5/1
  Delay4/1 -> Delay3/1
  Complex Multiplier/1(Out1) -> Delay2/1, Delay1/1
  Delay3/1 -> Delay17/1
  Delay1/1 -> Delay16/1
  Delay2/1 -> Complex Multiplier1/1(In1)
  Delay5/1 -> Complex Multiplier1/2(In2)
  Delay7/1 -> Delay18/1
  Delay17/1 -> Delay11/1
  Delay16/1 -> Delay9/1
  Complex Multiplier1/1(Out1) -> Delay10/1
  Delay10/1 -> Delay15/1, Complex Multiplier2/1(In1)
  Delay18/1 -> Delay12/1
  Delay11/1 -> Delay13/1
  Delay9/1 -> Delay14/1
  Complex Multiplier2/1(Out1) -> Delay27/1
  Delay12/1 -> Complex Multiplier2/2(In2)
  Delay13/1 -> Delay24/1
  Delay14/1 -> Delay25/1
  Delay25/1 -> Delay33/1
  Delay15/1 -> Delay26/1
  Delay24/1 -> Delay32/1
  Delay26/1 -> Delay34/1
  Delay27/1 -> Delay35/1
  Delay33/1 -> Gain/1(In1)
  Delay34/1 -> Delay20/1
  Delay35/1 -> Gain1/1(In1)
  Delay19/1 -> Delay28/1
  Gain/1(Out1) -> Delay29/1
  Delay20/1 -> Delay30/1
  Delay28/1 -> Multiport Switch/2
  Gain1/1(Out1) -> Delay31/1
  Delay29/1 -> Multiport Switch/3
  Delay30/1 -> Multiport Switch/4
  Delay31/1 -> Multiport Switch/5
  Delay36/1 -> dataOut/1

== system gm_soc_dvbs2_fpga/DVBS2/DVBS2 TxRx/DVB-S2 HDL Receiver/Synchronizer and PL Header Decoder/PL Header Recovery/PL Frame Demultiplexer ==
  endOfSOFIn : Inport  OutDataTypeStr=boolean  PortDimensions=1  SampleTime=2.5e-07
  validIn : Inport  Port=2  OutDataTypeStr=boolean  PortDimensions=1  SampleTime=2.5e-07
  Compare To Constant : simulink/Logic and Bit Operations/Compare To Constant  relop=<=  const=config.PLSCLength - 1  OutDataTypeStr=boolean
  Delay : Delay  DelayLength=64
  Delay{1..3,5..8,10..13} (11 alike) : Delay  DelayLength=1
  HDL Counter : hdlsllib/Sources/HDL Counter  CountType=Free running  CountInit=0  CountStep=1  CountMax=25  CountFromType=Initial value  CountFrom=0  CountResetPort=on  CountLoadPort=off  CountEnbPort=on  CountDirPort=off  CountHitOutputPort=off  CountDataType=Unsigned  CountWordLen=32  CountFracLen=0  CountSampTime=1
  Logical Operator : Logic  Inputs=3  AllPortsSameDT=off  OutDataTypeStr=boolean
  Logical Operator1 : Logic  AllPortsSameDT=off  OutDataTypeStr=boolean
  Logical Operator2 : Logic  Operator=NOT  AllPortsSameDT=off  OutDataTypeStr=boolean
  Unit Delay Enabled Synchronous : hdlsllib/Discrete/Unit Delay Enabled Synchronous  InitialCondition=0.0  SampleTime=-1
  hValid : Outport  SampleTime=2.5e-07
  dValid : Outport  Port=2  SampleTime=2.5e-07
  endOfPLSC : Outport  Port=3  SampleTime=2.5e-07
  wires:
  endOfSOFIn/1 -> Unit Delay Enabled Synchronous/2, Unit Delay Enabled Synchronous/1, Delay/1, HDL Counter/1
  Delay/1 -> Delay5/1
  Delay1/1 -> Logical Operator/2
  validIn/1 -> Delay2/1, HDL Counter/2
  Delay3/1 -> Logical Operator/1
  Unit Delay Enabled Synchronous/1 -> Delay3/1
  HDL Counter/1 -> Compare To Constant/1
  Delay5/1 -> Delay10/1
  Compare To Constant/1 -> Delay1/1
  Delay10/1 -> Delay13/1
  Delay2/1 -> Delay8/1, Logical Operator/3
  Delay13/1 -> endOfPLSC/1
  Logical Operator/1 -> Delay7/1, Delay6/1
  Delay6/1 -> Logical Operator2/1
  Delay7/1 -> Delay11/1
  Logical Operator2/1 -> Logical Operator1/1
  Delay8/1 -> Logical Operator1/2
  Delay11/1 -> hValid/1
  Logical Operator1/1 -> Delay12/1
  Delay12/1 -> dValid/1

== system gm_soc_dvbs2_fpga/DVBS2/DVBS2 TxRx/DVB-S2 HDL Receiver/Synchronizer and PL Header Decoder/PL Header Recovery/PL Header Decoder ==
  dataIn : Inport  OutDataTypeStr=fixdt(1, 18, 13)  PortDimensions=1  SampleTime=2.5e-07
      settings: SignalType=complex
  hasPilots : Inport  Port=2  OutDataTypeStr=boolean  PortDimensions=1  SampleTime=2.5e-07
  endOfSOF : Inport  Port=3  OutDataTypeStr=boolean  PortDimensions=1  SampleTime=2.5e-07
  validIn : Inport  Port=4  OutDataTypeStr=boolean  PortDimensions=1  SampleTime=2.5e-07
  Bit Flipping and Averaging : Subsystem
  Constant : Constant  Value="fi(0,1,18,13,\"hex\",\"00000 + 00000 i\")"  OutDataTypeStr=fixdt(1, 18, 13)  SampleTime=2.5e-07
  Delay{1..4} (4 alike) : Delay  DelayLength=double(1)  InitialCondition=0  SampleTime=2.5e-07
  Delay5 : Delay  DelayLength=double(10)  InitialCondition=0  SampleTime=2.5e-07
  Delay6 : Delay  DelayLength=double(4)  InitialCondition=0  SampleTime=2.5e-07
  Extract Bits2 : simulink/Logic and Bit Operations/Extract Bits  bitsToExtract=Range of bits  numBits=8  bitIdxRange=[1 5]  outScalingMode=Treat bit field as an integer
  ML Decoder : Subsystem
  PLSC Descrambler : Subsystem
  Switch : Switch  Criteria=u2 ~= 0  Threshold="fi(0,0,1,0,\"hex\",\"0\")"  OutDataTypeStr=fixdt(1, 18, 13)  SampleTime=2.5e-07  SaturateOnIntegerOverflow=off  InputSameDT=off
  dtc1_Extract Bits3 : DataTypeConversion  OutDataTypeStr=fixdt(0, 1, 0)  SampleTime=2.5e-07  SaturateOnIntegerOverflow=off  RndMeth=Floor
  pi/2 BPSK Soft Bit Generator : Subsystem
  modcod : Outport  SampleTime=2.5e-07
  FECFrame : Outport  Port=2  SampleTime=2.5e-07
  wires:
  Switch/1 -> PLSC Descrambler/1(dataIn)
  endOfSOF/1 -> Delay1/1
  dataIn/1 -> Delay3/1
  hasPilots/1 -> Delay4/1
  validIn/1 -> Delay2/1
  pi/2 BPSK Soft Bit Generator/3(validOut) -> Bit Flipping and Averaging/3(validIn)
  Delay3/1 -> Switch/1
  Delay2/1 -> PLSC Descrambler/3(validIn), Switch/2
  Constant/1 -> Switch/3
  Delay1/1 -> PLSC Descrambler/2(resetIn)
  Delay4/1 -> Delay5/1
  PLSC Descrambler/1(dataOut) -> pi/2 BPSK Soft Bit Generator/1(dataIn)
  pi/2 BPSK Soft Bit Generator/4(resetOut) -> Bit Flipping and Averaging/4(resetIn)
  PLSC Descrambler/2(indexIndicator) -> pi/2 BPSK Soft Bit Generator/2(indexIndicatorIn)
  PLSC Descrambler/3(validOut) -> pi/2 BPSK Soft Bit Generator/3(validIn)
  pi/2 BPSK Soft Bit Generator/2(indexIndicatorOut) -> Bit Flipping and Averaging/2(indexIndicater)
  PLSC Descrambler/4(resetOut) -> pi/2 BPSK Soft Bit Generator/4(resetIn)
  pi/2 BPSK Soft Bit Generator/1(dataOut) -> Bit Flipping and Averaging/1(dataIn)
  Delay5/1 -> Delay6/1
  Delay6/1 -> Bit Flipping and Averaging/5(hasPilots)
  Bit Flipping and Averaging/1(dataOut) -> ML Decoder/1(dataIn)
  dtc1_Extract Bits3/1 -> FECFrame/1
  Bit Flipping and Averaging/2(validOut) -> ML Decoder/2(PLSCValid32)
  Bit Flipping and Averaging/3(resetOut) -> ML Decoder/3(reset)
  ML Decoder/1(bits6Out) -> dtc1_Extract Bits3/1, Extract Bits2/1
  Extract Bits2/1 -> modcod/1

== system gm_soc_dvbs2_fpga/DVBS2/DVBS2 TxRx/DVB-S2 HDL Receiver/Synchronizer and PL Header Decoder/Source Encoding/MATLAB Function ==
  In : Inport  OutDataTypeStr=fixdt(0, 5, 0)  PortDimensions=1  SampleTime=2.5e-07
  MATLAB Function : MATLAB Function  TreatAsAtomicUnit=on
  MATLAB Function_term1 : Terminator
  t : Constant  Value=double(0)  OutDataTypeStr=boolean  SampleTime=2.5e-07
  out : Outport  SampleTime=2.5e-07
  isdummy : Outport  Port=2  SampleTime=2.5e-07
  wires:
  MATLAB Function/1(out) -> out/1
  t/1 -> isdummy/1
  In/1 -> MATLAB Function/1(In)
  MATLAB Function/2(isdummy) -> MATLAB Function_term1/1

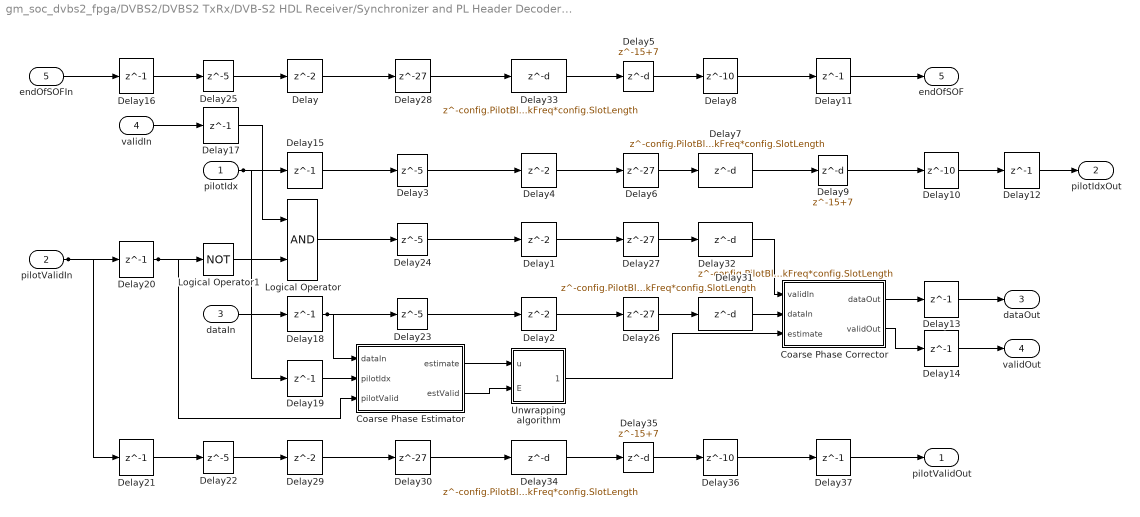
== system gm_soc_dvbs2_fpga/DVBS2/DVBS2 TxRx/DVB-S2 HDL Receiver/Synchronizer and PL Header Decoder/Time Frequency and Coarse Phase Synchronizer/Coarse Phase Synchronizer ==
  pilotIdx : Inport  OutDataTypeStr=fixdt(0, 11, 0)  PortDimensions=1  SampleTime=2.5e-07
  pilotValidIn : Inport  Port=2  OutDataTypeStr=boolean  PortDimensions=1  SampleTime=2.5e-07
  dataIn : Inport  Port=3  OutDataTypeStr=fixdt(1, 18, 13)  PortDimensions=1  SampleTime=2.5e-07
      settings: SignalType=complex
  validIn : Inport  Port=4  OutDataTypeStr=boolean  PortDimensions=1  SampleTime=2.5e-07
  endOfSOFIn : Inport  Port=5  OutDataTypeStr=boolean  PortDimensions=1  SampleTime=2.5e-07
  Coarse Phase Corrector : Subsystem
  Coarse Phase Estimator : Subsystem
  Delay{,1..2,4,29} (5 alike) : Delay
  Delay10 : Delay  DelayLength=10  InitialCondition=0
  Delay{11..21,37} (12 alike) : Delay  DelayLength=1  InitialCondition=0
  Delay{3,22..25} (5 alike) : Delay  DelayLength=5  InitialCondition=0
  Delay{6,26..28,30} (5 alike) : Delay  DelayLength=27
  Delay{7,31..34} (5 alike) : Delay  DelayLength=config.PilotBlkFreq*config.SlotLength
  Delay35 : Delay  DelayLength=15+7
  Delay36 : Delay  DelayLength=10  InitialCondition=0
  Delay5 : Delay  DelayLength=15+7
  Delay8 : Delay  DelayLength=10  InitialCondition=0
  Delay9 : Delay  DelayLength=15+7
  Logical Operator : Logic  AllPortsSameDT=off  OutDataTypeStr=boolean
  Logical Operator1 : Logic  Operator=NOT  AllPortsSameDT=off  OutDataTypeStr=boolean
  Unwrapping algorithm : Subsystem
  pilotValidOut : Outport  SampleTime=2.5e-07
  pilotIdxOut : Outport  Port=2  SampleTime=2.5e-07
  dataOut : Outport  Port=3  SampleTime=2.5e-07
  validOut : Outport  Port=4  SampleTime=2.5e-07
  endOfSOF : Outport  Port=5  SampleTime=2.5e-07
  wires:
  Delay33/1 -> Delay5/1
  endOfSOFIn/1 -> Delay16/1
  Delay34/1 -> Delay35/1
  validIn/1 -> Delay17/1
  Delay36/1 -> Delay37/1
  pilotValidIn/1 -> Delay21/1, Delay20/1
  Delay25/1 -> Delay/1
  Delay21/1 -> Delay22/1
  Delay16/1 -> Delay25/1
  Delay17/1 -> Logical Operator/1
  Delay20/1 -> Coarse Phase Estimator/3(pilotValid), Logical Operator1/1
  Delay3/1 -> Delay4/1
  pilotIdx/1 -> Delay19/1, Delay15/1
  Delay6/1 -> Delay7/1
  Logical Operator1/1 -> Logical Operator/2
  Delay35/1 -> Delay36/1
  dataIn/1 -> Delay18/1
  Delay22/1 -> Delay29/1
  Delay/1 -> Delay28/1
  Delay15/1 -> Delay3/1
  Delay5/1 -> Delay8/1
  Logical Operator/1 -> Delay24/1
  Delay18/1 -> Delay23/1, Coarse Phase Estimator/1(dataIn)
  Delay19/1 -> Coarse Phase Estimator/2(pilotIdx)
  Delay29/1 -> Delay30/1
  Delay28/1 -> Delay33/1
  Delay24/1 -> Delay1/1
  Delay23/1 -> Delay2/1
  Coarse Phase Estimator/1(estimate) -> Unwrapping algorithm/1(u)
  Coarse Phase Estimator/2(estValid) -> Unwrapping algorithm/2(E)
  Delay30/1 -> Delay34/1
  Delay4/1 -> Delay6/1
  Delay1/1 -> Delay27/1
  Delay2/1 -> Delay26/1
  Delay31/1 -> Coarse Phase Corrector/2(dataIn)
  Unwrapping algorithm/1(estimate) -> Coarse Phase Corrector/3(estimate)
  Delay27/1 -> Delay32/1
  Delay26/1 -> Delay31/1
  Delay8/1 -> Delay11/1
  Delay7/1 -> Delay9/1
  Delay32/1 -> Coarse Phase Corrector/1(validIn)
  Delay11/1 -> endOfSOF/1
  Delay9/1 -> Delay10/1
  Coarse Phase Corrector/1(dataOut) -> Delay13/1
  Coarse Phase Corrector/2(validOut) -> Delay14/1
  Delay37/1 -> pilotValidOut/1
  Delay10/1 -> Delay12/1
  Delay13/1 -> dataOut/1
  Delay14/1 -> validOut/1
  Delay12/1 -> pilotIdxOut/1

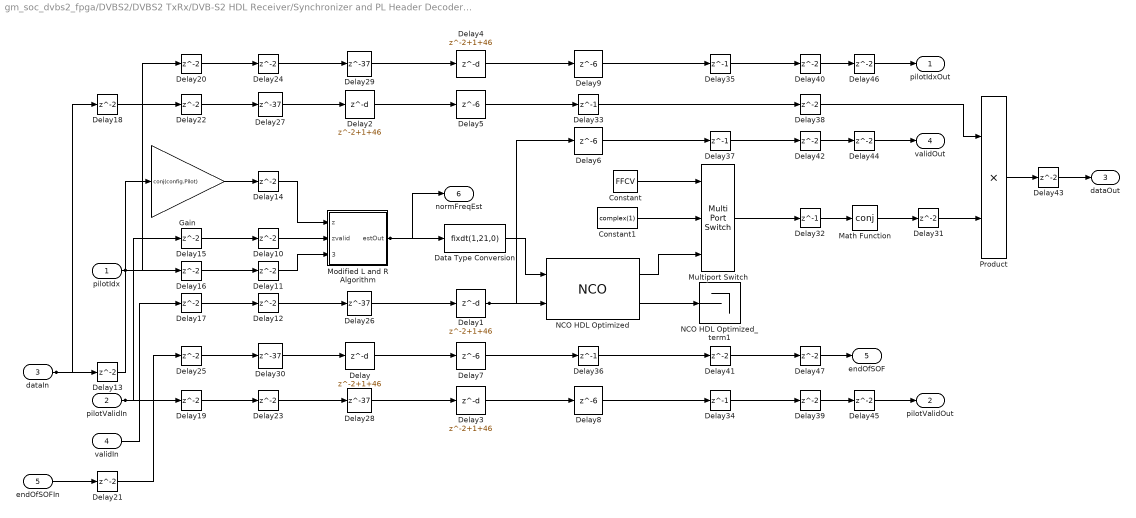
== system gm_soc_dvbs2_fpga/DVBS2/DVBS2 TxRx/DVB-S2 HDL Receiver/Synchronizer and PL Header Decoder/Time Frequency and Coarse Phase Synchronizer/Fine Frequency Synchronizer ==
  pilotIdx : Inport  OutDataTypeStr=fixdt(0, 11, 0)  PortDimensions=1  SampleTime=2.5e-07
  pilotValidIn : Inport  Port=2  OutDataTypeStr=boolean  PortDimensions=1  SampleTime=2.5e-07
  dataIn : Inport  Port=3  OutDataTypeStr=fixdt(1, 18, 13)  PortDimensions=1  SampleTime=2.5e-07
      settings: SignalType=complex
  validIn : Inport  Port=4  OutDataTypeStr=boolean  PortDimensions=1  SampleTime=2.5e-07
  endOfSOFIn : Inport  Port=5  OutDataTypeStr=boolean  PortDimensions=1  SampleTime=2.5e-07
  Constant : Constant  Value=FFCV  OutDataTypeStr=boolean  SampleTime=-1
  Constant1 : Constant  Value=complex(1)  OutDataTypeStr=fixdt(1, 16, 14)  SampleTime=-1
  Data Type Conversion : DataTypeConversion  OutDataTypeStr=fixdt(1,21,0)  ConvertRealWorld=Stored Integer (SI)  SaturateOnIntegerOverflow=off  RndMeth=Floor
  Delay{,1..4} (5 alike) : Delay  DelayLength=2+1+46
  Delay{10..25,31,38..47} (27 alike) : Delay
  Delay{26..30} (5 alike) : Delay  DelayLength=37
  Delay{32..37} (6 alike) : Delay  DelayLength=1
  Delay{5..9} (5 alike) : Delay  DelayLength=6
  Gain : Gain  Gain=conj(config.Pilot)  OutDataTypeStr=fixdt(1, 18, 13)
      mask init:
      | Simulink.suppressDiagnostic(gcb, 'SimulinkFixedPoint:util:fxpParameterPrecisionLoss');
  Math Function : Math  Operator=conj  OutDataTypeStr=fixdt(1, 16, 14)
  Modified L and R Algorithm : Subsystem
  Multiport Switch : MultiPortSwitch  DataPortOrder=Zero-based contiguous  Inputs=2  zeroidx=on  OutDataTypeStr=fixdt(1, 16, 14)  SaturateOnIntegerOverflow=off  InputSameDT=off
  NCO HDL Optimized : dsphdlsigops2/NCO  PhaseIncrementSource=Input port  PhaseIncrement=100  PhaseOffsetSource=Property  PhaseOffset=0  DitherSource=None  NumDitherBits=4  SamplesPerFrame=1  LUTCompress=off  ResetAction=off  Waveform=Complex exponential  PhasePort=off  SimulateUsing=Code generation  AccumulatorWL=21  PhaseQuantization=on  NumQuantizerAccumulatorBits=14  OutputDataType=Binary point scaling  OutputWL=16  OutputFL=14
  NCO HDL Optimized_term1 : Terminator
  Product : Product  OutDataTypeStr=fixdt(1, 18, 13)
  pilotIdxOut : Outport  SampleTime=2.5e-07
  pilotValidOut : Outport  Port=2  SampleTime=2.5e-07
  dataOut : Outport  Port=3  SampleTime=2.5e-07
  validOut : Outport  Port=4  SampleTime=2.5e-07
  endOfSOF : Outport  Port=5  SampleTime=2.5e-07
  normFreqEst : Outport  Port=6  SampleTime=2.5e-07
  wires:
  Delay19/1 -> Delay23/1
  Delay13/1 -> Gain/1
  Delay15/1 -> Delay10/1
  pilotIdx/1 -> Delay20/1, Delay16/1
  Delay20/1 -> Delay24/1
  dataIn/1 -> Delay18/1, Delay13/1
  Modified L and R Algorithm/1(estOut) -> normFreqEst/1, Data Type Conversion/1
  endOfSOFIn/1 -> Delay21/1
  Delay21/1 -> Delay25/1
  Delay14/1 -> Modified L and R Algorithm/1(z)
  validIn/1 -> Delay17/1
  pilotValidIn/1 -> Delay19/1, Delay15/1
  Delay12/1 -> Delay26/1
  Delay18/1 -> Delay22/1
  Delay22/1 -> Delay27/1
  Gain/1 -> Delay14/1
  Delay10/1 -> Modified L and R Algorithm/2(zvalid)
  Delay16/1 -> Delay11/1
  Delay11/1 -> Modified L and R Algorithm/3(pilotIdx)
  Delay17/1 -> Delay12/1
  Delay4/1 -> Delay9/1
  Delay25/1 -> Delay30/1
  Delay39/1 -> Delay45/1
  Delay24/1 -> Delay29/1
  Delay41/1 -> Delay47/1
  Delay27/1 -> Delay2/1
  Delay30/1 -> Delay/1
  Delay38/1 -> Product/1
  Delay23/1 -> Delay28/1
  Delay29/1 -> Delay4/1
  Delay2/1 -> Delay5/1
  Delay40/1 -> Delay46/1
  Delay26/1 -> Delay1/1
  Delay/1 -> Delay7/1
  Delay28/1 -> Delay3/1
  Multiport Switch/1 -> Delay32/1
  Delay5/1 -> Delay33/1
  Data Type Conversion/1 -> NCO HDL Optimized/1
  Constant/1 -> Multiport Switch/1
  Delay1/1 -> Delay6/1, NCO HDL Optimized/2
  Delay7/1 -> Delay36/1
  Delay3/1 -> Delay8/1
  Delay9/1 -> Delay35/1
  Delay33/1 -> Delay38/1
  Product/1 -> Delay43/1
  Math Function/1 -> Delay31/1
  Delay6/1 -> Delay37/1
  Constant1/1 -> Multiport Switch/2
  Delay45/1 -> pilotValidOut/1
  NCO HDL Optimized/1 -> Multiport Switch/3
  NCO HDL Optimized/2 -> NCO HDL Optimized_term1/1
  Delay36/1 -> Delay41/1
  Delay8/1 -> Delay34/1
  Delay35/1 -> Delay40/1
  Delay37/1 -> Delay42/1
  Delay34/1 -> Delay39/1
  Delay42/1 -> Delay44/1
  Delay32/1 -> Math Function/1
  Delay47/1 -> endOfSOF/1
  Delay46/1 -> pilotIdxOut/1
  Delay44/1 -> validOut/1
  Delay31/1 -> Product/2
  Delay43/1 -> dataOut/1
